simulink model "IMC_FNM"  (R2014a)
settings: Solver=ode45  StartTime=0.0  StopTime=1900  RelTol=1e-3
settings Model: Creator=Imaculada  LastModifiedBy=Imaculada

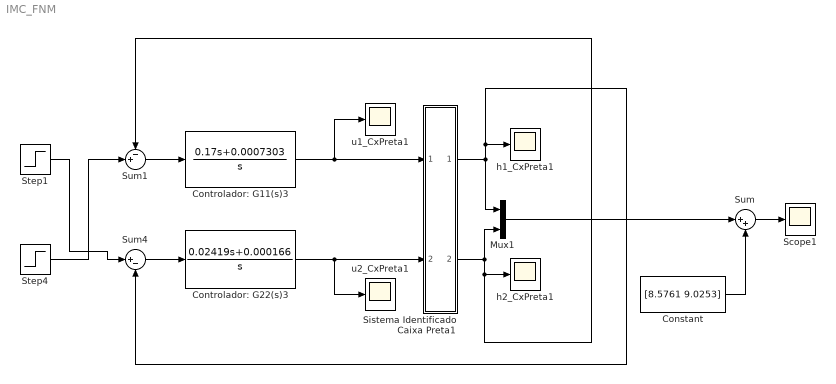
== system IMC_FNM ==
  Constant : Constant  Value=[8.5761 9.0253]
  Controlador: G11(s)3 : TransferFcn  Numerator=[0.17 0.0007303]  Denominator=[1 0]
  Controlador: G22(s)3 : TransferFcn  Numerator=[0.02419 0.000166]  Denominator=[1 0]
  Mux1 : Mux  Inputs=2
  Scope1 : Scope
      settings: SaveName=Simulado
  Sistema Identificado Caixa Preta1 : Subsystem
  Step1 : Step  Time=300  SampleTime=0
  Step4 : Step  Time=1100  SampleTime=0
  Sum : Sum  Inputs=|++
  Sum1 : Sum  Inputs=-+|
  Sum4 : Sum  Inputs=|+-
  h1_CxPreta1 : Scope
      settings: SaveName=ScopeData6
  h2_CxPreta1 : Scope
      settings: SaveName=ScopeData7
  u1_CxPreta1 : Scope
      settings: SaveName=ScopeData8
  u2_CxPreta1 : Scope
      settings: SaveName=ScopeData9
  wires:
  Sistema Identificado Caixa Preta1/1(h1) -> Mux1/1, h1_CxPreta1/1, Sum4/2
  Sistema Identificado Caixa Preta1/2(h2) -> Sum1/1, h2_CxPreta1/1, Mux1/2
  Controlador: G22(s)3/1 -> Sistema Identificado Caixa Preta1/2(u2), u2_CxPreta1/1
  Controlador: G11(s)3/1 -> Sistema Identificado Caixa Preta1/1(u1), u1_CxPreta1/1
  Sum1/1 -> Controlador: G11(s)3/1
  Sum4/1 -> Controlador: G22(s)3/1
  Sum/1 -> Scope1/1
  Mux1/1 -> Sum/1
  Constant/1 -> Sum/2
  Step4/1 -> Sum1/2
  Step1/1 -> Sum4/1

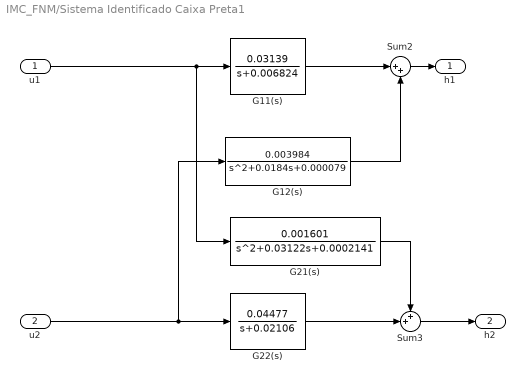
== system IMC_FNM/Sistema Identificado Caixa Preta1 ==
  u1 : Inport
  u2 : Inport  Port=2
  G11(s) : TransferFcn  Numerator=[0 0.03139]  Denominator=[1 0.006824]
  G12(s) : TransferFcn  Numerator=[0 0 0.003984]  Denominator=[1 0.0184 0.000079]
  G21(s) : TransferFcn  Numerator=[0 0 0.001601]  Denominator=[1 0.03122 0.0002141]
  G22(s) : TransferFcn  Numerator=[0 0.04477]  Denominator=[1 0.02106]
  Sum2 : Sum  Inputs=|++
  Sum3 : Sum  Inputs=++|
  h1 : Outport
  h2 : Outport  Port=2
  wires:
  G11(s)/1 -> Sum2/1
  G22(s)/1 -> Sum3/2
  G12(s)/1 -> Sum2/2
  G21(s)/1 -> Sum3/1
  Sum2/1 -> h1/1
  Sum3/1 -> h2/1
  u1/1 -> G21(s)/1, G11(s)/1
  u2/1 -> G12(s)/1, G22(s)/1
